simulink model "Microgrid_W"  (R2020a)
settings: Solver=ode15s  StartTime=0  StopTime=1440*1  MaxStep=1  RelTol=1e-3
libraries: simulink x4214, powerlib x685, simulink_extras x28, Microgrid_Library x18, powerlib_meascontrol x12
(part 1 of 48)
settings Model: Creator=burmesdani  LastModifiedBy=danie
settings SolverCC: ZeroCrossAlgorithm=Adaptive
settings DataIOCC: ReturnWorkspaceOutputs=off
settings DebuggingCC: MaxConsecutiveZCsMsg=none  ArithmeticOperatorsInVariantConditions=warning
settings SFSimCC: SimUseLocalCustomCode=off  CustomCodeUndefinedFunction=UseInterfaceOnly
settings RTWCC: RTWUseLocalCustomCode=off
settings CodeAppCC: StateflowObjectComments=on
settings SimscapeCC: SimscapeNormalizeSystem=off

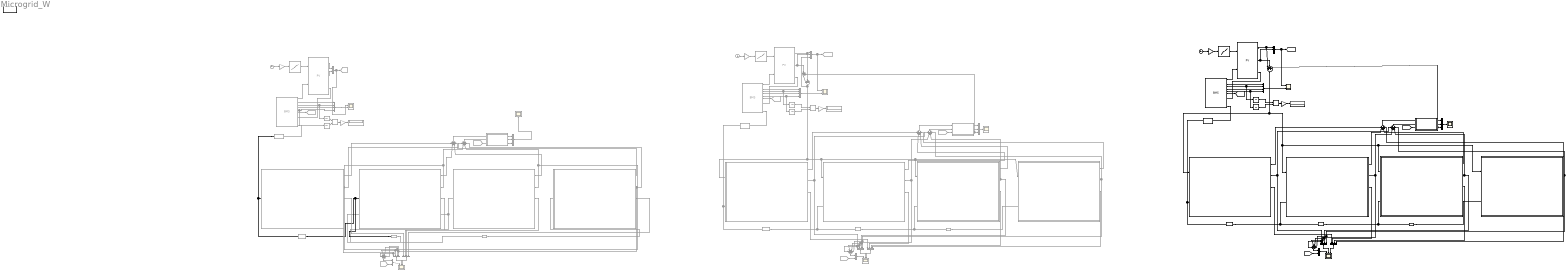
== system Microgrid_W ==
  note: Uncontrolled Microgrid
  note: Controlled Microgrid
  note: Controlled Microgrid
  1-D Lookup Table1 : Lookup_n-D  NumberOfTableDimensions=1  BreakpointsForDimension1=[ 0 1 2 3 4 5 6 7 8 9 10 11 12 13 14 15 16 17 18 19 20 21 22 23 24 25 26 27 28 29 30 31 32 33 34 35 36 37 38 39 40 41 42 43 44 45 46 47 48 49 50 51 52 53 54 55 56 57 58 59 60 61 62 63 64 65 66 67 68 69 70 71 72 73 74 75 76 77 78 79 80 81 82 83 84 85 86 87 88 89 90 91 92 93 94 95 96 97 98 99 100 101 102 103 104 105 106 107 108 109 110 111 112 113 114 115 116 117 118 119 120 121 122 123 124 125 126 127 128 129 130 131 132 133 134 135 136 137 138 139 140 141 142 143 144 145 146 147 148 149 150 151 152 153 154 155 156 157 158 159 160 161 162 163 164 165 166 167 ]  Table=|  InternalRulePriority=Speed  RndMeth=Simplest  InputSameDT=on
      | [ 0 0 0 0 0 0 0 0 24 102 216 265 347 180 457 139 14 0 0 0 0 0 0 0 0 0 0 0 0 0 0 3 102 438 606 521 454 674 419 211 67 0 0 0 0 0 0 0 0 0 0 0 0 0 0 0 20 56 105 60 86 80 111 69 23 0 0 0 0 0 0 0 0 0 0 0 0 0 0 0 20 59 207 329 494 326 573 325 86 0 0 0 0 0 0 0 0 0 0 0 0 0 0 3 79 461 545 698 753 631 556 256 120 0 0 0 0 0 0 0 0 0 0 0 0 0 0 0 23 289 555 185 105 97 116 180 25 0 0 0 0 0 0 0 0 0 0 0 0 0 0 0 26 66 128 161 217 251 160 48 40 0 0 0 0 0 0 0 
      | ]
  1-D Lookup Table2 : Lookup_n-D  Commented=on  NumberOfTableDimensions=1  BreakpointsForDimension1=[ 0 1 2 3 4 5 6 7 8 9 10 11 12 13 14 15 16 17 18 19 20 21 22 23 24 25 26 27 28 29 30 31 32 33 34 35 36 37 38 39 40 41 42 43 44 45 46 47 48 49 50 51 52 53 54 55 56 57 58 59 60 61 62 63 64 65 66 67 68 69 70 71 72 73 74 75 76 77 78 79 80 81 82 83 84 85 86 87 88 89 90 91 92 93 94 95 96 97 98 99 100 101 102 103 104 105 106 107 108 109 110 111 112 113 114 115 116 117 118 119 120 121 122 123 124 125 126 127 128 129 130 131 132 133 134 135 136 137 138 139 140 141 142 143 144 145 146 147 148 149 150 151 152 153 154 155 156 157 158 159 160 161 162 163 164 165 166 167 ]  Table=|  InternalRulePriority=Speed  RndMeth=Simplest  InputSameDT=on
      | [ 0 0 0 0 0 0 0 0 24 102 216 265 347 180 457 139 14 0 0 0 0 0 0 0 0 0 0 0 0 0 0 3 102 438 606 521 454 674 419 211 67 0 0 0 0 0 0 0 0 0 0 0 0 0 0 0 20 56 105 60 86 80 111 69 23 0 0 0 0 0 0 0 0 0 0 0 0 0 0 0 20 59 207 329 494 326 573 325 86 0 0 0 0 0 0 0 0 0 0 0 0 0 0 3 79 461 545 698 753 631 556 256 120 0 0 0 0 0 0 0 0 0 0 0 0 0 0 0 23 289 555 185 105 97 116 180 25 0 0 0 0 0 0 0 0 0 0 0 0 0 0 0 26 66 128 161 217 251 160 48 40 0 0 0 0 0 0 0 
      | ]
  1-D Lookup Table3 : Lookup_n-D  Commented=on  NumberOfTableDimensions=1  BreakpointsForDimension1=[ 0 1 2 3 4 5 6 7 8 9 10 11 12 13 14 15 16 17 18 19 20 21 22 23 24 25 26 27 28 29 30 31 32 33 34 35 36 37 38 39 40 41 42 43 44 45 46 47 48 49 50 51 52 53 54 55 56 57 58 59 60 61 62 63 64 65 66 67 68 69 70 71 72 73 74 75 76 77 78 79 80 81 82 83 84 85 86 87 88 89 90 91 92 93 94 95 96 97 98 99 100 101 102 103 104 105 106 107 108 109 110 111 112 113 114 115 116 117 118 119 120 121 122 123 124 125 126 127 128 129 130 131 132 133 134 135 136 137 138 139 140 141 142 143 144 145 146 147 148 149 150 151 152 153 154 155 156 157 158 159 160 161 162 163 164 165 166 167 ]  Table=|  InternalRulePriority=Speed  RndMeth=Simplest  InputSameDT=on
      | [ 0 0 0 0 0 0 0 0 24 102 216 265 347 180 457 139 14 0 0 0 0 0 0 0 0 0 0 0 0 0 0 3 102 438 606 521 454 674 419 211 67 0 0 0 0 0 0 0 0 0 0 0 0 0 0 0 20 56 105 60 86 80 111 69 23 0 0 0 0 0 0 0 0 0 0 0 0 0 0 0 20 59 207 329 494 326 573 325 86 0 0 0 0 0 0 0 0 0 0 0 0 0 0 3 79 461 545 698 753 631 556 256 120 0 0 0 0 0 0 0 0 0 0 0 0 0 0 0 23 289 555 185 105 97 116 180 25 0 0 0 0 0 0 0 0 0 0 0 0 0 0 0 26 66 128 161 217 251 160 48 40 0 0 0 0 0 0 0 
      | ]
  161m1 : Microgrid_Library/Line  l=161
  161m2 : Microgrid_Library/Line  Commented=on  l=161
  161m3 : Microgrid_Library/Line  Commented=on  l=161
  47m1 : Microgrid_Library/Line  l=47
  47m2 : Microgrid_Library/Line  Commented=on  l=47
  47m3 : Microgrid_Library/Line  Commented=on  l=47
  58m1 : Microgrid_Library/Line  l=58
  58m2 : Microgrid_Library/Line  Commented=on  l=58
  58m3 : Microgrid_Library/Line  Commented=on  l=58
  60m1 : Microgrid_Library/Line  l=60
  60m2 : Microgrid_Library/Line  Commented=on  l=60
  60m3 : Microgrid_Library/Line  Commented=on  l=60
  BMS1 : Microgrid_Library/BMS  v=240  c=460
  BMS2 : Microgrid_Library/BMS  Commented=on  v=240  c=460
  BMS3 : Microgrid_Library/BMS  Commented=on  v=240  c=460
  Clock1 : Clock
  Clock2 : Clock  Commented=on
  Clock3 : Clock  Commented=on
  Divide1 : Product  Inputs=*/
  Divide2 : Product  Commented=on  Inputs=*/
  Divide3 : Product  Commented=on  Inputs=*/
  From1 : From  Commented=on  GotoTag=PV
  From3 : From  Commented=on  GotoTag=bat_sup
  From4 : From  Commented=on  GotoTag=PV_MUX
  From5 : From  Commented=on  GotoTag=bat_sup
  Gain1 : Gain  Gain=1/60
  Gain2 : Gain  Gain=100
  Gain3 : Gain  Commented=on  Gain=1/60
  Gain4 : Gain  Commented=on  Gain=100
  Gain5 : Gain  Commented=on  Gain=1/60
  Gain6 : Gain  Commented=on  Gain=100
  Goto2 : Goto  Commented=on  GotoTag=PV
  Goto3 : Goto  Commented=on  GotoTag=bat_sup
  Goto4 : Goto  Commented=on  GotoTag=PV_MUX
  Goto5 : Goto  Commented=on  GotoTag=bat_sup
  House 2 W1 : Subsystem  AncestorBlock=Microgrid_Library/House 2 W  mask{V=240, t=60, K_L1_W=40, K_L1_On_1=63000, K_L1_Off_1=72600, K_L1_On_2=0, K_L1_Off_2=0, Dishwasher_W=1200, Dishwasher_On=72000, Fridge_W=150, T_Initial=1.9, T_Low=1, T_High=2.4, Jug_W=1500, Jug_On_1=25200, Jug_On_2=64200, Jug_On_3=0, Toaster_W=900, Toaster_On_1=23400, Toaster_On_2=27120, N_Elements=4, Oven_On_1=63600, Oven_Off_1=67200, Shower_On_a=21720, Shower_L_a=240, Shower_On_b=23640, Shower_L_b=300, Shower_On_c=0, Shower_L_c=0, K_L3_W=60, K_L3_On_1=21480, K_L3_Off_1=22140, K_L3_On_2=23580, K_L3_Off_2=24780, HW_W=2000, M=177, D=0.488, L=1.72, Ti=7, Ta=20, T_Low_WH=58, T_High_WH=61, Clock_1_W=5, Lamp_1_W=18, L1_On_1=79740, L1_Off_1=83040, L1_On_2=0, L1_Off_2=0, K_L4_W=24, K_L4_On_1=21000, K_L4_Off_1=27360, Clock_2_W=6, Lamp_2_W=24, L2_On_1=26820, L2_Off_1=29160, L2_On_2=73800, L2_Off_2=76800, K_L5_W=40, K_L5_On_1=28800, K_L5_Off_1=30240, K_L5_On_2=72300, K_L5_Off_2=83880, Phone_C_1_W=3, Phone_C_1_On_a=0, Phone_C_1_Off_a=35700, Phone_C_1_On_b=76800, Phone_C_1_Off_b=86400, Phone_C_2_W=7, Phone_C_2_On_a=0, Phone_C_2_Off_a=35760, Phone_C_2_On_b=76800, Phone_C_2_Off_b=86400, Phone_C_3_W=5, Phone_C_3_On_a=0, Phone_C_3_Off_a=35700, Phone_C_3_On_b=77040, Phone_C_3_Off_b=86400, Laptop_C_1_W=55, Laptop_C_1_On_a=76800, Laptop_C_1_Off_a=86400, Laptop_C_2_W=65, Laptop_C_2_On_a=0, Laptop_C_2_Off_a=28500, Laptop_C_2_On_b=77160, Laptop_C_2_Off_b=86400, Lamp_3_W=60, L3_On_1=21600, L3_Off_1=27000, L3_On_2=62760, L3_Off_2=83220, K_L6_W=60, K_L6_On_1=68400, K_L6_Off_1=70200, Heater_W=1800, Heater_On_1=62040, Heater_Off_1=68640, Stereo_W=100, Stereo_On_1=42480, Stereo_Off_1=58200, TV_W=500, TV_On_1=21900, TV_Off_1=26580, TV_On_2=63000, TV_Off_2=73200}
      mask prompts: V "Voltage"; t "Time"; K_L1_W "Light_1_W"; K_L1_On_1 "Light_1_On_a"; K_L1_Off_1 "Light_1_Off_a"; K_L1_On_2 "Light_1_On_b"; K_L1_Off_2 "Light_1_Off_b"; T_Initial "Fridge_Initial_Temp"; T_Low "Fridge_T_Low"; T_High "Fridge_T_High"; N_Elements "Oven_#_Elements"; Shower_L_a "Shower_Length_a"; Shower_L_b "Shower_Length_b"; Shower_L_c "Shower_Length_c"; K_L3_W "Light_3_W"; K_L3_On_1 "Light_3_On_a"; K_L3_Off_1 "Light_3_Off_a"; K_L3_On_2 "Light_3_On_b"; K_L3_Off_2 "Light_3_Off_b"; M "Mass of water"; D "HW_Diameter"; L "HW_Length"; Ti "Inlet Temp"; Ta "Ambient Temp"; L1_On_1 "Lamp_1_On_1"; L1_Off_1 "Lamp_1_Off_1"; L1_On_2 "Lamp_1_On_2"; L1_Off_2 "Lamp_1_Off_2"; K_L4_W "Light_4_W"; K_L4_On_1 "Light_4_On_a"; K_L4_Off_1 "Light_4_Off_a"; L2_On_1 "Lamp_2_On_1"; L2_Off_1 "Lamp_2_Off_1"; L2_On_2 "Lamp_2_On_2"; L2_Off_2 "Lamp_2_Off_2"; K_L5_W "Light_5_W"; K_L5_On_1 "Light_5_On_a"; K_L5_Off_1 "Light_5_Off_a"; K_L5_On_2 "Light_5_On_b"; K_L5_Off_2 "Light_5_Off_b"; L3_On_1 "Lamp_3_On_1"; L3_Off_1 "Lamp_3_Off_1"; L3_On_2 "Lamp_3_On_2"; L3_Off_2 "Lamp_3_Off_2"; K_L6_W "Light_6_W"; K_L6_On_1 "Light_6_On_a"; K_L6_Off_1 "Light_6_Off_a"
      mask DialogControl Container4 Prompt: House 1
      mask DialogControl Container10 Prompt: Kitchen
      mask DialogControl Container22 Prompt: Bathroom
      mask DialogControl Container20 Prompt: Bedroom 1
      mask DialogControl Container16 Prompt: Bedroom 2
      mask DialogControl Container11 Prompt: Lounge
      mask Display: image('house.jpg');
  House 2 W2 : Subsystem  Commented=on  AncestorBlock=Microgrid_Library/House 2 W  mask{V=240, t=60, K_L1_W=40, K_L1_On_1=63000, K_L1_Off_1=72600, K_L1_On_2=0, K_L1_Off_2=0, Dishwasher_W=1200, Dishwasher_On=72000, Fridge_W=150, T_Initial=1.9, T_Low=1, T_High=2.4, Jug_W=1500, Jug_On_1=25200, Jug_On_2=64200, Jug_On_3=0, Toaster_W=900, Toaster_On_1=23400, Toaster_On_2=27120, N_Elements=4, Oven_On_1=63600, Oven_Off_1=67200, Shower_On_a=21720, Shower_L_a=240, Shower_On_b=23640, Shower_L_b=300, Shower_On_c=0, Shower_L_c=0, K_L3_W=60, K_L3_On_1=21480, K_L3_Off_1=22140, K_L3_On_2=23580, K_L3_Off_2=24780, HW_W=2000, M=177, D=0.488, L=1.72, Ti=7, Ta=20, T_Low_WH=58, T_High_WH=61, Clock_1_W=5, Lamp_1_W=18, L1_On_1=79740, L1_Off_1=83040, L1_On_2=0, L1_Off_2=0, K_L4_W=24, K_L4_On_1=21000, K_L4_Off_1=27360, Clock_2_W=6, Lamp_2_W=24, L2_On_1=26820, L2_Off_1=29160, L2_On_2=73800, L2_Off_2=76800, K_L5_W=40, K_L5_On_1=28800, K_L5_Off_1=30240, K_L5_On_2=72300, K_L5_Off_2=83880, Phone_C_1_W=3, Phone_C_1_On_a=0, Phone_C_1_Off_a=35700, Phone_C_1_On_b=76800, Phone_C_1_Off_b=86400, Phone_C_2_W=7, Phone_C_2_On_a=0, Phone_C_2_Off_a=35760, Phone_C_2_On_b=76800, Phone_C_2_Off_b=86400, Phone_C_3_W=5, Phone_C_3_On_a=0, Phone_C_3_Off_a=35700, Phone_C_3_On_b=77040, Phone_C_3_Off_b=86400, Laptop_C_1_W=55, Laptop_C_1_On_a=76800, Laptop_C_1_Off_a=86400, Laptop_C_2_W=65, Laptop_C_2_On_a=0, Laptop_C_2_Off_a=28500, Laptop_C_2_On_b=77160, Laptop_C_2_Off_b=86400, Lamp_3_W=60, L3_On_1=21600, L3_Off_1=27000, L3_On_2=62760, L3_Off_2=83220, K_L6_W=60, K_L6_On_1=68400, K_L6_Off_1=70200, Heater_W=1800, Heater_On_1=62040, Heater_Off_1=68640, Stereo_W=100, Stereo_On_1=42480, Stereo_Off_1=58200, TV_W=500, TV_On_1=21900, TV_Off_1=26580, TV_On_2=63000, TV_Off_2=73200}
      mask prompts: V "Voltage"; t "Time"; K_L1_W "Light_1_W"; K_L1_On_1 "Light_1_On_a"; K_L1_Off_1 "Light_1_Off_a"; K_L1_On_2 "Light_1_On_b"; K_L1_Off_2 "Light_1_Off_b"; T_Initial "Fridge_Initial_Temp"; T_Low "Fridge_T_Low"; T_High "Fridge_T_High"; N_Elements "Oven_#_Elements"; Shower_L_a "Shower_Length_a"; Shower_L_b "Shower_Length_b"; Shower_L_c "Shower_Length_c"; K_L3_W "Light_3_W"; K_L3_On_1 "Light_3_On_a"; K_L3_Off_1 "Light_3_Off_a"; K_L3_On_2 "Light_3_On_b"; K_L3_Off_2 "Light_3_Off_b"; M "Mass of water"; D "HW_Diameter"; L "HW_Length"; Ti "Inlet Temp"; Ta "Ambient Temp"; L1_On_1 "Lamp_1_On_1"; L1_Off_1 "Lamp_1_Off_1"; L1_On_2 "Lamp_1_On_2"; L1_Off_2 "Lamp_1_Off_2"; K_L4_W "Light_4_W"; K_L4_On_1 "Light_4_On_a"; K_L4_Off_1 "Light_4_Off_a"; L2_On_1 "Lamp_2_On_1"; L2_Off_1 "Lamp_2_Off_1"; L2_On_2 "Lamp_2_On_2"; L2_Off_2 "Lamp_2_Off_2"; K_L5_W "Light_5_W"; K_L5_On_1 "Light_5_On_a"; K_L5_Off_1 "Light_5_Off_a"; K_L5_On_2 "Light_5_On_b"; K_L5_Off_2 "Light_5_Off_b"; L3_On_1 "Lamp_3_On_1"; L3_Off_1 "Lamp_3_Off_1"; L3_On_2 "Lamp_3_On_2"; L3_Off_2 "Lamp_3_Off_2"; K_L6_W "Light_6_W"; K_L6_On_1 "Light_6_On_a"; K_L6_Off_1 "Light_6_Off_a"
      mask DialogControl Container4 Prompt: House 1
      mask DialogControl Container10 Prompt: Kitchen
      mask DialogControl Container22 Prompt: Bathroom
      mask DialogControl Container20 Prompt: Bedroom 1
      mask DialogControl Container16 Prompt: Bedroom 2
      mask DialogControl Container11 Prompt: Lounge
      mask Display: image('house.jpg');
  House 2 W3 : Subsystem  Commented=on  AncestorBlock=Microgrid_Library/House 2 W  mask{V=240, t=60, K_L1_W=40, K_L1_On_1=63000, K_L1_Off_1=72600, K_L1_On_2=0, K_L1_Off_2=0, Dishwasher_W=1200, Dishwasher_On=72000, Fridge_W=150, T_Initial=1.9, T_Low=1, T_High=2.4, Jug_W=1500, Jug_On_1=25200, Jug_On_2=64200, Jug_On_3=0, Toaster_W=900, Toaster_On_1=23400, Toaster_On_2=27120, N_Elements=4, Oven_On_1=63600, Oven_Off_1=67200, Shower_On_a=21720, Shower_L_a=240, Shower_On_b=23640, Shower_L_b=300, Shower_On_c=0, Shower_L_c=0, K_L3_W=60, K_L3_On_1=21480, K_L3_Off_1=22140, K_L3_On_2=23580, K_L3_Off_2=24780, HW_W=2000, M=177, D=0.488, L=1.72, Ti=7, Ta=20, T_Low_WH=58, T_High_WH=61, Clock_1_W=5, Lamp_1_W=18, L1_On_1=79740, L1_Off_1=83040, L1_On_2=0, L1_Off_2=0, K_L4_W=24, K_L4_On_1=21000, K_L4_Off_1=27360, Clock_2_W=6, Lamp_2_W=24, L2_On_1=26820, L2_Off_1=29160, L2_On_2=73800, L2_Off_2=76800, K_L5_W=40, K_L5_On_1=28800, K_L5_Off_1=30240, K_L5_On_2=72300, K_L5_Off_2=83880, Phone_C_1_W=3, Phone_C_1_On_a=0, Phone_C_1_Off_a=35700, Phone_C_1_On_b=76800, Phone_C_1_Off_b=86400, Phone_C_2_W=7, Phone_C_2_On_a=0, Phone_C_2_Off_a=35760, Phone_C_2_On_b=76800, Phone_C_2_Off_b=86400, Phone_C_3_W=5, Phone_C_3_On_a=0, Phone_C_3_Off_a=35700, Phone_C_3_On_b=77040, Phone_C_3_Off_b=86400, Laptop_C_1_W=55, Laptop_C_1_On_a=76800, Laptop_C_1_Off_a=86400, Laptop_C_2_W=65, Laptop_C_2_On_a=0, Laptop_C_2_Off_a=28500, Laptop_C_2_On_b=77160, Laptop_C_2_Off_b=86400, Lamp_3_W=60, L3_On_1=21600, L3_Off_1=27000, L3_On_2=62760, L3_Off_2=83220, K_L6_W=60, K_L6_On_1=68400, K_L6_Off_1=70200, Heater_W=1800, Heater_On_1=62040, Heater_Off_1=68640, Stereo_W=100, Stereo_On_1=42480, Stereo_Off_1=58200, TV_W=500, TV_On_1=21900, TV_Off_1=26580, TV_On_2=63000, TV_Off_2=73200}
      mask prompts: V "Voltage"; t "Time"; K_L1_W "Light_1_W"; K_L1_On_1 "Light_1_On_a"; K_L1_Off_1 "Light_1_Off_a"; K_L1_On_2 "Light_1_On_b"; K_L1_Off_2 "Light_1_Off_b"; T_Initial "Fridge_Initial_Temp"; T_Low "Fridge_T_Low"; T_High "Fridge_T_High"; N_Elements "Oven_#_Elements"; Shower_L_a "Shower_Length_a"; Shower_L_b "Shower_Length_b"; Shower_L_c "Shower_Length_c"; K_L3_W "Light_3_W"; K_L3_On_1 "Light_3_On_a"; K_L3_Off_1 "Light_3_Off_a"; K_L3_On_2 "Light_3_On_b"; K_L3_Off_2 "Light_3_Off_b"; M "Mass of water"; D "HW_Diameter"; L "HW_Length"; Ti "Inlet Temp"; Ta "Ambient Temp"; L1_On_1 "Lamp_1_On_1"; L1_Off_1 "Lamp_1_Off_1"; L1_On_2 "Lamp_1_On_2"; L1_Off_2 "Lamp_1_Off_2"; K_L4_W "Light_4_W"; K_L4_On_1 "Light_4_On_a"; K_L4_Off_1 "Light_4_Off_a"; L2_On_1 "Lamp_2_On_1"; L2_Off_1 "Lamp_2_Off_1"; L2_On_2 "Lamp_2_On_2"; L2_Off_2 "Lamp_2_Off_2"; K_L5_W "Light_5_W"; K_L5_On_1 "Light_5_On_a"; K_L5_Off_1 "Light_5_Off_a"; K_L5_On_2 "Light_5_On_b"; K_L5_Off_2 "Light_5_Off_b"; L3_On_1 "Lamp_3_On_1"; L3_Off_1 "Lamp_3_Off_1"; L3_On_2 "Lamp_3_On_2"; L3_Off_2 "Lamp_3_Off_2"; K_L6_W "Light_6_W"; K_L6_On_1 "Light_6_On_a"; K_L6_Off_1 "Light_6_Off_a"
      mask DialogControl Container4 Prompt: House 1
      mask DialogControl Container10 Prompt: Kitchen
      mask DialogControl Container22 Prompt: Bathroom
      mask DialogControl Container20 Prompt: Bedroom 1
      mask DialogControl Container16 Prompt: Bedroom 2
      mask DialogControl Container11 Prompt: Lounge
      mask Display: image('house.jpg');
  House 3 W1 : Subsystem  AncestorBlock=Microgrid_Library/House 3 W  mask{V=240, t=60, K_L1_W=24, K_L1_On_1=21600, K_L1_Off_1=26580, K_L1_On_2=63000, K_L1_Off_2=68400, K_L2_W=60, K_L2_On_1=63000, K_L2_Off_1=68400, Fridge_W=200, T_Initial=1.5, T_Low=1.5, T_High=2.65, Jug_W=2000, Jug_On_1=21720, Jug_On_2=43560, Jug_On_3=73800, Toaster_W=1200, Toaster_On_1=25260, Toaster_On_2=28920, N_Elements=1, Oven_On_1=58680, Oven_Off_1=68760, Shower_On_a=70440, Shower_L_a=360, Shower_On_b=76740, Shower_L_b=180, Shower_On_c=81000, Shower_L_c=180, K_L3_W=80, K_L3_On_1=70200, K_L3_Off_1=70800, K_L3_On_2=76320, K_L3_Off_2=81300, HW_W=3000, M=250, D=0.58, L=1.56, Ti=7, Ta=20, T_Low_WH=59, T_High_WH=61, Clock_1_W=6, Lamp_1_W=18, L1_On_1=71400, L1_Off_1=81120, L1_On_2=0, L1_Off_2=0, K_L4_W=60, K_L4_On_1=69600, K_L4_Off_1=71400, Clock_2_W=4, Lamp_2_W=24, L2_On_1=84120, L2_Off_1=86880, L2_On_2=0, L2_Off_2=0, K_L5_W=40, K_L5_On_1=25320, K_L5_Off_1=28980, K_L5_On_2=81000, K_L5_Off_2=84180, Phone_C_1_W=7, Phone_C_1_On_a=0, Phone_C_1_Off_a=27300, Phone_C_1_On_b=79200, Phone_C_1_Off_b=86400, Phone_C_2_W=6, Phone_C_2_On_a=0, Phone_C_2_Off_a=27300, Phone_C_2_On_b=79200, Phone_C_2_Off_b=86400, Phone_C_3_W=5, Phone_C_3_On_a=0, Phone_C_3_Off_a=0, Phone_C_3_On_b=0, Phone_C_3_Off_b=0, Laptop_C_1_W=1, Laptop_C_1_On_a=0, Laptop_C_1_Off_a=0, Laptop_C_2_W=45, Laptop_C_2_On_a=0, Laptop_C_2_Off_a=6000, Laptop_C_2_On_b=66600, Laptop_C_2_Off_b=86400, Lamp_3_W=40, L3_On_1=24900, L3_Off_1=30600, L3_On_2=72000, L3_Off_2=81000, K_L6_W=60, K_L6_On_1=68760, K_L6_Off_1=71520, Heater_W=1500, Heater_On_1=64800, Heater_Off_1=78000, Stereo_W=1, Stereo_On_1=0, Stereo_Off_1=0, TV_W=150, TV_On_1=25200, TV_Off_1=28800, TV_On_2=72240, TV_Off_2=81000}
      mask prompts: V "Voltage"; t "Time"; K_L1_W "Light_1_W"; K_L1_On_1 "Light_1_On_a"; K_L1_Off_1 "Light_1_Off_a"; K_L1_On_2 "Light_1_On_b"; K_L1_Off_2 "Light_1_Off_b"; K_L2_W "Light_2_W"; K_L2_On_1 "Light_2_On_a"; K_L2_Off_1 "Light_2_Off_a"; T_Initial "Fridge_Initial_Temp"; T_Low "Fridge_T_Low"; T_High "Fridge_T_High"; N_Elements "Oven_#_Elements"; Shower_L_a "Shower_Length_a"; Shower_L_b "Shower_Length_b"; Shower_L_c "Shower_Length_c"; K_L3_W "Light_3_W"; K_L3_On_1 "Light_3_On_a"; K_L3_Off_1 "Light_3_Off_a"; K_L3_On_2 "Light_3_On_b"; K_L3_Off_2 "Light_3_Off_b"; M "Mass of water"; D "HW_Diameter"; L "HW_Length"; Ti "Inlet Temp"; Ta "Ambient Temp"; L1_On_1 "Lamp_1_On_1"; L1_Off_1 "Lamp_1_Off_1"; L1_On_2 "Lamp_1_On_2"; L1_Off_2 "Lamp_1_Off_2"; K_L4_W "Light_4_W"; K_L4_On_1 "Light_4_On_a"; K_L4_Off_1 "Light_4_Off_a"; L2_On_1 "Lamp_2_On_1"; L2_Off_1 "Lamp_2_Off_1"; L2_On_2 "Lamp_2_On_2"; L2_Off_2 "Lamp_2_Off_2"; K_L5_W "Light_5_W"; K_L5_On_1 "Light_5_On_a"; K_L5_Off_1 "Light_5_Off_a"; K_L5_On_2 "Light_5_On_b"; K_L5_Off_2 "Light_5_Off_b"; L3_On_1 "Lamp_3_On_1"; L3_Off_1 "Lamp_3_Off_1"; L3_On_2 "Lamp_3_On_2"; L3_Off_2 "Lamp_3_Off_2"; K_L6_W "Light_6_W"; K_L6_On_1 "Light_6_On_a"; K_L6_Off_1 "Light_6_Off_a"
      mask DialogControl Container4 Prompt: House 1
      mask DialogControl Container10 Prompt: Kitchen
      mask DialogControl Container22 Prompt: Bathroom
      mask DialogControl Container20 Prompt: Bedroom 1
      mask DialogControl Container16 Prompt: Bedroom 2
      mask DialogControl Container11 Prompt: Lounge
      mask Display: image('house.jpg');
  House 3 W2 : Subsystem  Commented=on  AncestorBlock=Microgrid_Library/House 3 W  mask{V=240, t=60, K_L1_W=24, K_L1_On_1=21600, K_L1_Off_1=26580, K_L1_On_2=63000, K_L1_Off_2=68400, K_L2_W=60, K_L2_On_1=63000, K_L2_Off_1=68400, Fridge_W=200, T_Initial=1.5, T_Low=1.5, T_High=2.65, Jug_W=2000, Jug_On_1=21720, Jug_On_2=43560, Jug_On_3=73800, Toaster_W=1200, Toaster_On_1=25260, Toaster_On_2=28920, N_Elements=1, Oven_On_1=58680, Oven_Off_1=68760, Shower_On_a=70440, Shower_L_a=360, Shower_On_b=76740, Shower_L_b=180, Shower_On_c=81000, Shower_L_c=180, K_L3_W=80, K_L3_On_1=70200, K_L3_Off_1=70800, K_L3_On_2=76320, K_L3_Off_2=81300, HW_W=3000, M=250, D=0.58, L=1.56, Ti=7, Ta=20, T_Low_WH=59, T_High_WH=61, Clock_1_W=6, Lamp_1_W=18, L1_On_1=71400, L1_Off_1=81120, L1_On_2=0, L1_Off_2=0, K_L4_W=60, K_L4_On_1=69600, K_L4_Off_1=71400, Clock_2_W=4, Lamp_2_W=24, L2_On_1=84120, L2_Off_1=86880, L2_On_2=0, L2_Off_2=0, K_L5_W=40, K_L5_On_1=25320, K_L5_Off_1=28980, K_L5_On_2=81000, K_L5_Off_2=84180, Phone_C_1_W=7, Phone_C_1_On_a=0, Phone_C_1_Off_a=27300, Phone_C_1_On_b=79200, Phone_C_1_Off_b=86400, Phone_C_2_W=6, Phone_C_2_On_a=0, Phone_C_2_Off_a=27300, Phone_C_2_On_b=79200, Phone_C_2_Off_b=86400, Phone_C_3_W=5, Phone_C_3_On_a=0, Phone_C_3_Off_a=0, Phone_C_3_On_b=0, Phone_C_3_Off_b=0, Laptop_C_1_W=1, Laptop_C_1_On_a=0, Laptop_C_1_Off_a=0, Laptop_C_2_W=45, Laptop_C_2_On_a=0, Laptop_C_2_Off_a=6000, Laptop_C_2_On_b=66600, Laptop_C_2_Off_b=86400, Lamp_3_W=40, L3_On_1=24900, L3_Off_1=30600, L3_On_2=72000, L3_Off_2=81000, K_L6_W=60, K_L6_On_1=68760, K_L6_Off_1=71520, Heater_W=1500, Heater_On_1=64800, Heater_Off_1=78000, Stereo_W=1, Stereo_On_1=0, Stereo_Off_1=0, TV_W=150, TV_On_1=25200, TV_Off_1=28800, TV_On_2=72240, TV_Off_2=81000}
      mask prompts: V "Voltage"; t "Time"; K_L1_W "Light_1_W"; K_L1_On_1 "Light_1_On_a"; K_L1_Off_1 "Light_1_Off_a"; K_L1_On_2 "Light_1_On_b"; K_L1_Off_2 "Light_1_Off_b"; K_L2_W "Light_2_W"; K_L2_On_1 "Light_2_On_a"; K_L2_Off_1 "Light_2_Off_a"; T_Initial "Fridge_Initial_Temp"; T_Low "Fridge_T_Low"; T_High "Fridge_T_High"; N_Elements "Oven_#_Elements"; Shower_L_a "Shower_Length_a"; Shower_L_b "Shower_Length_b"; Shower_L_c "Shower_Length_c"; K_L3_W "Light_3_W"; K_L3_On_1 "Light_3_On_a"; K_L3_Off_1 "Light_3_Off_a"; K_L3_On_2 "Light_3_On_b"; K_L3_Off_2 "Light_3_Off_b"; M "Mass of water"; D "HW_Diameter"; L "HW_Length"; Ti "Inlet Temp"; Ta "Ambient Temp"; L1_On_1 "Lamp_1_On_1"; L1_Off_1 "Lamp_1_Off_1"; L1_On_2 "Lamp_1_On_2"; L1_Off_2 "Lamp_1_Off_2"; K_L4_W "Light_4_W"; K_L4_On_1 "Light_4_On_a"; K_L4_Off_1 "Light_4_Off_a"; L2_On_1 "Lamp_2_On_1"; L2_Off_1 "Lamp_2_Off_1"; L2_On_2 "Lamp_2_On_2"; L2_Off_2 "Lamp_2_Off_2"; K_L5_W "Light_5_W"; K_L5_On_1 "Light_5_On_a"; K_L5_Off_1 "Light_5_Off_a"; K_L5_On_2 "Light_5_On_b"; K_L5_Off_2 "Light_5_Off_b"; L3_On_1 "Lamp_3_On_1"; L3_Off_1 "Lamp_3_Off_1"; L3_On_2 "Lamp_3_On_2"; L3_Off_2 "Lamp_3_Off_2"; K_L6_W "Light_6_W"; K_L6_On_1 "Light_6_On_a"; K_L6_Off_1 "Light_6_Off_a"
      mask DialogControl Container4 Prompt: House 1
      mask DialogControl Container10 Prompt: Kitchen
      mask DialogControl Container22 Prompt: Bathroom
      mask DialogControl Container20 Prompt: Bedroom 1
      mask DialogControl Container16 Prompt: Bedroom 2
      mask DialogControl Container11 Prompt: Lounge
      mask Display: image('house.jpg');
  House 3 W3 : Subsystem  Commented=on  AncestorBlock=Microgrid_Library/House 3 W  mask{V=240, t=60, K_L1_W=24, K_L1_On_1=21600, K_L1_Off_1=26580, K_L1_On_2=63000, K_L1_Off_2=68400, K_L2_W=60, K_L2_On_1=63000, K_L2_Off_1=68400, Fridge_W=200, T_Initial=1.5, T_Low=1.5, T_High=2.65, Jug_W=2000, Jug_On_1=21720, Jug_On_2=43560, Jug_On_3=73800, Toaster_W=1200, Toaster_On_1=25260, Toaster_On_2=28920, N_Elements=1, Oven_On_1=58680, Oven_Off_1=68760, Shower_On_a=70440, Shower_L_a=360, Shower_On_b=76740, Shower_L_b=180, Shower_On_c=81000, Shower_L_c=180, K_L3_W=80, K_L3_On_1=70200, K_L3_Off_1=70800, K_L3_On_2=76320, K_L3_Off_2=81300, HW_W=3000, M=250, D=0.58, L=1.56, Ti=7, Ta=20, T_Low_WH=59, T_High_WH=61, Clock_1_W=6, Lamp_1_W=18, L1_On_1=71400, L1_Off_1=81120, L1_On_2=0, L1_Off_2=0, K_L4_W=60, K_L4_On_1=69600, K_L4_Off_1=71400, Clock_2_W=4, Lamp_2_W=24, L2_On_1=84120, L2_Off_1=86880, L2_On_2=0, L2_Off_2=0, K_L5_W=40, K_L5_On_1=25320, K_L5_Off_1=28980, K_L5_On_2=81000, K_L5_Off_2=84180, Phone_C_1_W=7, Phone_C_1_On_a=0, Phone_C_1_Off_a=27300, Phone_C_1_On_b=79200, Phone_C_1_Off_b=86400, Phone_C_2_W=6, Phone_C_2_On_a=0, Phone_C_2_Off_a=27300, Phone_C_2_On_b=79200, Phone_C_2_Off_b=86400, Phone_C_3_W=5, Phone_C_3_On_a=0, Phone_C_3_Off_a=0, Phone_C_3_On_b=0, Phone_C_3_Off_b=0, Laptop_C_1_W=1, Laptop_C_1_On_a=0, Laptop_C_1_Off_a=0, Laptop_C_2_W=45, Laptop_C_2_On_a=0, Laptop_C_2_Off_a=6000, Laptop_C_2_On_b=66600, Laptop_C_2_Off_b=86400, Lamp_3_W=40, L3_On_1=24900, L3_Off_1=30600, L3_On_2=72000, L3_Off_2=81000, K_L6_W=60, K_L6_On_1=68760, K_L6_Off_1=71520, Heater_W=1500, Heater_On_1=64800, Heater_Off_1=78000, Stereo_W=1, Stereo_On_1=0, Stereo_Off_1=0, TV_W=150, TV_On_1=25200, TV_Off_1=28800, TV_On_2=72240, TV_Off_2=81000}
      mask prompts: V "Voltage"; t "Time"; K_L1_W "Light_1_W"; K_L1_On_1 "Light_1_On_a"; K_L1_Off_1 "Light_1_Off_a"; K_L1_On_2 "Light_1_On_b"; K_L1_Off_2 "Light_1_Off_b"; K_L2_W "Light_2_W"; K_L2_On_1 "Light_2_On_a"; K_L2_Off_1 "Light_2_Off_a"; T_Initial "Fridge_Initial_Temp"; T_Low "Fridge_T_Low"; T_High "Fridge_T_High"; N_Elements "Oven_#_Elements"; Shower_L_a "Shower_Length_a"; Shower_L_b "Shower_Length_b"; Shower_L_c "Shower_Length_c"; K_L3_W "Light_3_W"; K_L3_On_1 "Light_3_On_a"; K_L3_Off_1 "Light_3_Off_a"; K_L3_On_2 "Light_3_On_b"; K_L3_Off_2 "Light_3_Off_b"; M "Mass of water"; D "HW_Diameter"; L "HW_Length"; Ti "Inlet Temp"; Ta "Ambient Temp"; L1_On_1 "Lamp_1_On_1"; L1_Off_1 "Lamp_1_Off_1"; L1_On_2 "Lamp_1_On_2"; L1_Off_2 "Lamp_1_Off_2"; K_L4_W "Light_4_W"; K_L4_On_1 "Light_4_On_a"; K_L4_Off_1 "Light_4_Off_a"; L2_On_1 "Lamp_2_On_1"; L2_Off_1 "Lamp_2_Off_1"; L2_On_2 "Lamp_2_On_2"; L2_Off_2 "Lamp_2_Off_2"; K_L5_W "Light_5_W"; K_L5_On_1 "Light_5_On_a"; K_L5_Off_1 "Light_5_Off_a"; K_L5_On_2 "Light_5_On_b"; K_L5_Off_2 "Light_5_Off_b"; L3_On_1 "Lamp_3_On_1"; L3_Off_1 "Lamp_3_Off_1"; L3_On_2 "Lamp_3_On_2"; L3_Off_2 "Lamp_3_Off_2"; K_L6_W "Light_6_W"; K_L6_On_1 "Light_6_On_a"; K_L6_Off_1 "Light_6_Off_a"
      mask DialogControl Container4 Prompt: House 1
      mask DialogControl Container10 Prompt: Kitchen
      mask DialogControl Container22 Prompt: Bathroom
      mask DialogControl Container20 Prompt: Bedroom 1
      mask DialogControl Container16 Prompt: Bedroom 2
      mask DialogControl Container11 Prompt: Lounge
      mask Display: image('house.jpg');
  House 4 W1 : Subsystem  AncestorBlock=Microgrid_Library/House 4 W  mask{V=240, t=60, K_L1_W=60, K_L1_On_1=69180, K_L1_Off_1=70200, K_L1_On_2=0, K_L1_Off_2=0, K_L2_W=1, K_L2_On_1=0, K_L2_Off_1=0, Fridge_W=150, T_Initial=1, T_Low=1, T_High=3.6, Jug_W=1800, Jug_On_1=23760, Jug_On_2=79800, Jug_On_3=0, Toaster_W=1000, Toaster_On_1=21600, Toaster_On_2=0, N_Elements=2, Oven_On_1=69240, Oven_Off_1=70140, Shower_On_a=20040, Shower_L_a=180, Shower_On_b=0, Shower_L_b=0, Shower_On_c=0, Shower_L_c=0, K_L3_W=40, K_L3_On_1=19800, K_L3_Off_1=20400, K_L3_On_2=0, K_L3_Off_2=0, HW_W=2000, M=88, D=0.488, L=0.955, Ti=7, Ta=20, T_Low_WH=55, T_High_WH=59.5, Clock_1_W=0, Lamp_1_W=1, L1_On_1=0, L1_Off_1=0, L1_On_2=0, L1_Off_2=0, K_L4_W=1, K_L4_On_1=0, K_L4_Off_1=0, Clock_2_W=4, Lamp_2_W=40, L2_On_1=19680, L2_Off_1=21600, L2_On_2=82800, L2_Off_2=84600, K_L5_W=1, K_L5_On_1=0, K_L5_Off_1=0, K_L5_On_2=0, K_L5_Off_2=0, Phone_C_1_W=5, Phone_C_1_On_a=0, Phone_C_1_Off_a=27300, Phone_C_1_On_b=79200, Phone_C_1_Off_b=86400, Phone_C_2_W=0, Phone_C_2_On_a=0, Phone_C_2_Off_a=0, Phone_C_2_On_b=0, Phone_C_2_Off_b=0, Phone_C_3_W=0, Phone_C_3_On_a=0, Phone_C_3_Off_a=0, Phone_C_3_On_b=0, Phone_C_3_Off_b=0, Laptop_C_1_W=35, Laptop_C_1_On_a=63900, Laptop_C_1_Off_a=75600, Laptop_C_2_W=65, Laptop_C_2_On_a=0, Laptop_C_2_Off_a=21600, Laptop_C_2_On_b=66600, Laptop_C_2_Off_b=86400, Lamp_3_W=18, L3_On_1=66000, L3_Off_1=82800, L3_On_2=0, L3_Off_2=0, K_L6_W=40, K_L6_On_1=63000, K_L6_Off_1=66000, Heater_W=2000, Heater_On_1=65100, Heater_Off_1=82200, Stereo_W=100, Stereo_On_1=68640, Stereo_Off_1=70740, TV_W=300, TV_On_1=70800, TV_Off_1=82800, TV_On_2=0, TV_Off_2=0}
      mask prompts: V "Voltage"; t "Time"; K_L1_W "Light_1_W"; K_L1_On_1 "Light_1_On_a"; K_L1_Off_1 "Light_1_Off_a"; K_L1_On_2 "Light_1_On_b"; K_L1_Off_2 "Light_1_Off_b"; K_L2_W "Light_2_W"; K_L2_On_1 "Light_2_On_a"; K_L2_Off_1 "Light_2_Off_a"; T_Initial "Fridge_Initial_Temp"; T_Low "Fridge_T_Low"; T_High "Fridge_T_High"; N_Elements "Oven_#_Elements"; Shower_L_a "Shower_Length_a"; Shower_L_b "Shower_Length_b"; Shower_L_c "Shower_Length_c"; K_L3_W "Light_3_W"; K_L3_On_1 "Light_3_On_a"; K_L3_Off_1 "Light_3_Off_a"; K_L3_On_2 "Light_3_On_b"; K_L3_Off_2 "Light_3_Off_b"; M "Mass of water"; D "HW_Diameter"; L "HW_Length"; Ti "Inlet Temp"; Ta "Ambient Temp"; L1_On_1 "Lamp_1_On_1"; L1_Off_1 "Lamp_1_Off_1"; L1_On_2 "Lamp_1_On_2"; L1_Off_2 "Lamp_1_Off_2"; K_L4_W "Light_4_W"; K_L4_On_1 "Light_4_On_a"; K_L4_Off_1 "Light_4_Off_a"; L2_On_1 "Lamp_2_On_1"; L2_Off_1 "Lamp_2_Off_1"; L2_On_2 "Lamp_2_On_2"; L2_Off_2 "Lamp_2_Off_2"; K_L5_W "Light_5_W"; K_L5_On_1 "Light_5_On_a"; K_L5_Off_1 "Light_5_Off_a"; K_L5_On_2 "Light_5_On_b"; K_L5_Off_2 "Light_5_Off_b"; L3_On_1 "Lamp_3_On_1"; L3_Off_1 "Lamp_3_Off_1"; L3_On_2 "Lamp_3_On_2"; L3_Off_2 "Lamp_3_Off_2"; K_L6_W "Light_6_W"; K_L6_On_1 "Light_6_On_a"; K_L6_Off_1 "Light_6_Off_a"
      mask DialogControl Container4 Prompt: House 1
      mask DialogControl Container10 Prompt: Kitchen
      mask DialogControl Container22 Prompt: Bathroom
      mask DialogControl Container20 Prompt: Bedroom 1
      mask DialogControl Container16 Prompt: Bedroom 2
      mask DialogControl Container11 Prompt: Lounge
      mask Display: image('house.jpg');
  House 4 W2 : Subsystem  Commented=on  AncestorBlock=Microgrid_Library/House 4 W  mask{V=240, t=60, K_L1_W=60, K_L1_On_1=69180, K_L1_Off_1=70200, K_L1_On_2=0, K_L1_Off_2=0, K_L2_W=1, K_L2_On_1=0, K_L2_Off_1=0, Fridge_W=150, T_Initial=1, T_Low=1, T_High=3.6, Jug_W=1800, Jug_On_1=23760, Jug_On_2=79800, Jug_On_3=0, Toaster_W=1000, Toaster_On_1=21600, Toaster_On_2=0, N_Elements=2, Oven_On_1=69240, Oven_Off_1=70140, Shower_On_a=20040, Shower_L_a=180, Shower_On_b=0, Shower_L_b=0, Shower_On_c=0, Shower_L_c=0, K_L3_W=40, K_L3_On_1=19800, K_L3_Off_1=20400, K_L3_On_2=0, K_L3_Off_2=0, HW_W=2000, M=88, D=0.488, L=0.955, Ti=7, Ta=20, T_Low_WH=55, T_High_WH=59.5, Clock_1_W=0, Lamp_1_W=1, L1_On_1=0, L1_Off_1=0, L1_On_2=0, L1_Off_2=0, K_L4_W=1, K_L4_On_1=0, K_L4_Off_1=0, Clock_2_W=4, Lamp_2_W=40, L2_On_1=19680, L2_Off_1=21600, L2_On_2=82800, L2_Off_2=84600, K_L5_W=1, K_L5_On_1=0, K_L5_Off_1=0, K_L5_On_2=0, K_L5_Off_2=0, Phone_C_1_W=5, Phone_C_1_On_a=0, Phone_C_1_Off_a=27300, Phone_C_1_On_b=79200, Phone_C_1_Off_b=86400, Phone_C_2_W=0, Phone_C_2_On_a=0, Phone_C_2_Off_a=0, Phone_C_2_On_b=0, Phone_C_2_Off_b=0, Phone_C_3_W=0, Phone_C_3_On_a=0, Phone_C_3_Off_a=0, Phone_C_3_On_b=0, Phone_C_3_Off_b=0, Laptop_C_1_W=35, Laptop_C_1_On_a=63900, Laptop_C_1_Off_a=75600, Laptop_C_2_W=65, Laptop_C_2_On_a=0, Laptop_C_2_Off_a=21600, Laptop_C_2_On_b=66600, Laptop_C_2_Off_b=86400, Lamp_3_W=18, L3_On_1=66000, L3_Off_1=82800, L3_On_2=0, L3_Off_2=0, K_L6_W=40, K_L6_On_1=63000, K_L6_Off_1=66000, Heater_W=2000, Heater_On_1=65100, Heater_Off_1=82200, Stereo_W=100, Stereo_On_1=68640, Stereo_Off_1=70740, TV_W=300, TV_On_1=70800, TV_Off_1=82800, TV_On_2=0, TV_Off_2=0}
      mask prompts: V "Voltage"; t "Time"; K_L1_W "Light_1_W"; K_L1_On_1 "Light_1_On_a"; K_L1_Off_1 "Light_1_Off_a"; K_L1_On_2 "Light_1_On_b"; K_L1_Off_2 "Light_1_Off_b"; K_L2_W "Light_2_W"; K_L2_On_1 "Light_2_On_a"; K_L2_Off_1 "Light_2_Off_a"; T_Initial "Fridge_Initial_Temp"; T_Low "Fridge_T_Low"; T_High "Fridge_T_High"; N_Elements "Oven_#_Elements"; Shower_L_a "Shower_Length_a"; Shower_L_b "Shower_Length_b"; Shower_L_c "Shower_Length_c"; K_L3_W "Light_3_W"; K_L3_On_1 "Light_3_On_a"; K_L3_Off_1 "Light_3_Off_a"; K_L3_On_2 "Light_3_On_b"; K_L3_Off_2 "Light_3_Off_b"; M "Mass of water"; D "HW_Diameter"; L "HW_Length"; Ti "Inlet Temp"; Ta "Ambient Temp"; L1_On_1 "Lamp_1_On_1"; L1_Off_1 "Lamp_1_Off_1"; L1_On_2 "Lamp_1_On_2"; L1_Off_2 "Lamp_1_Off_2"; K_L4_W "Light_4_W"; K_L4_On_1 "Light_4_On_a"; K_L4_Off_1 "Light_4_Off_a"; L2_On_1 "Lamp_2_On_1"; L2_Off_1 "Lamp_2_Off_1"; L2_On_2 "Lamp_2_On_2"; L2_Off_2 "Lamp_2_Off_2"; K_L5_W "Light_5_W"; K_L5_On_1 "Light_5_On_a"; K_L5_Off_1 "Light_5_Off_a"; K_L5_On_2 "Light_5_On_b"; K_L5_Off_2 "Light_5_Off_b"; L3_On_1 "Lamp_3_On_1"; L3_Off_1 "Lamp_3_Off_1"; L3_On_2 "Lamp_3_On_2"; L3_Off_2 "Lamp_3_Off_2"; K_L6_W "Light_6_W"; K_L6_On_1 "Light_6_On_a"; K_L6_Off_1 "Light_6_Off_a"
      mask DialogControl Container4 Prompt: House 1
      mask DialogControl Container10 Prompt: Kitchen
      mask DialogControl Container22 Prompt: Bathroom
      mask DialogControl Container20 Prompt: Bedroom 1
      mask DialogControl Container16 Prompt: Bedroom 2
      mask DialogControl Container11 Prompt: Lounge
      mask Display: image('house.jpg');
  House 4 W3 : Subsystem  Commented=on  AncestorBlock=Microgrid_Library/House 4 W  mask{V=240, t=60, K_L1_W=60, K_L1_On_1=69180, K_L1_Off_1=70200, K_L1_On_2=0, K_L1_Off_2=0, K_L2_W=1, K_L2_On_1=0, K_L2_Off_1=0, Fridge_W=150, T_Initial=1, T_Low=1, T_High=3.6, Jug_W=1800, Jug_On_1=23760, Jug_On_2=79800, Jug_On_3=0, Toaster_W=1000, Toaster_On_1=21600, Toaster_On_2=0, N_Elements=2, Oven_On_1=69240, Oven_Off_1=70140, Shower_On_a=20040, Shower_L_a=180, Shower_On_b=0, Shower_L_b=0, Shower_On_c=0, Shower_L_c=0, K_L3_W=40, K_L3_On_1=19800, K_L3_Off_1=20400, K_L3_On_2=0, K_L3_Off_2=0, HW_W=2000, M=88, D=0.488, L=0.955, Ti=7, Ta=20, T_Low_WH=55, T_High_WH=59.5, Clock_1_W=0, Lamp_1_W=1, L1_On_1=0, L1_Off_1=0, L1_On_2=0, L1_Off_2=0, K_L4_W=1, K_L4_On_1=0, K_L4_Off_1=0, Clock_2_W=4, Lamp_2_W=40, L2_On_1=19680, L2_Off_1=21600, L2_On_2=82800, L2_Off_2=84600, K_L5_W=1, K_L5_On_1=0, K_L5_Off_1=0, K_L5_On_2=0, K_L5_Off_2=0, Phone_C_1_W=5, Phone_C_1_On_a=0, Phone_C_1_Off_a=27300, Phone_C_1_On_b=79200, Phone_C_1_Off_b=86400, Phone_C_2_W=0, Phone_C_2_On_a=0, Phone_C_2_Off_a=0, Phone_C_2_On_b=0, Phone_C_2_Off_b=0, Phone_C_3_W=0, Phone_C_3_On_a=0, Phone_C_3_Off_a=0, Phone_C_3_On_b=0, Phone_C_3_Off_b=0, Laptop_C_1_W=35, Laptop_C_1_On_a=63900, Laptop_C_1_Off_a=75600, Laptop_C_2_W=65, Laptop_C_2_On_a=0, Laptop_C_2_Off_a=21600, Laptop_C_2_On_b=66600, Laptop_C_2_Off_b=86400, Lamp_3_W=18, L3_On_1=66000, L3_Off_1=82800, L3_On_2=0, L3_Off_2=0, K_L6_W=40, K_L6_On_1=63000, K_L6_Off_1=66000, Heater_W=2000, Heater_On_1=65100, Heater_Off_1=82200, Stereo_W=100, Stereo_On_1=68640, Stereo_Off_1=70740, TV_W=300, TV_On_1=70800, TV_Off_1=82800, TV_On_2=0, TV_Off_2=0}
      mask prompts: V "Voltage"; t "Time"; K_L1_W "Light_1_W"; K_L1_On_1 "Light_1_On_a"; K_L1_Off_1 "Light_1_Off_a"; K_L1_On_2 "Light_1_On_b"; K_L1_Off_2 "Light_1_Off_b"; K_L2_W "Light_2_W"; K_L2_On_1 "Light_2_On_a"; K_L2_Off_1 "Light_2_Off_a"; T_Initial "Fridge_Initial_Temp"; T_Low "Fridge_T_Low"; T_High "Fridge_T_High"; N_Elements "Oven_#_Elements"; Shower_L_a "Shower_Length_a"; Shower_L_b "Shower_Length_b"; Shower_L_c "Shower_Length_c"; K_L3_W "Light_3_W"; K_L3_On_1 "Light_3_On_a"; K_L3_Off_1 "Light_3_Off_a"; K_L3_On_2 "Light_3_On_b"; K_L3_Off_2 "Light_3_Off_b"; M "Mass of water"; D "HW_Diameter"; L "HW_Length"; Ti "Inlet Temp"; Ta "Ambient Temp"; L1_On_1 "Lamp_1_On_1"; L1_Off_1 "Lamp_1_Off_1"; L1_On_2 "Lamp_1_On_2"; L1_Off_2 "Lamp_1_Off_2"; K_L4_W "Light_4_W"; K_L4_On_1 "Light_4_On_a"; K_L4_Off_1 "Light_4_Off_a"; L2_On_1 "Lamp_2_On_1"; L2_Off_1 "Lamp_2_Off_1"; L2_On_2 "Lamp_2_On_2"; L2_Off_2 "Lamp_2_Off_2"; K_L5_W "Light_5_W"; K_L5_On_1 "Light_5_On_a"; K_L5_Off_1 "Light_5_Off_a"; K_L5_On_2 "Light_5_On_b"; K_L5_Off_2 "Light_5_Off_b"; L3_On_1 "Lamp_3_On_1"; L3_Off_1 "Lamp_3_Off_1"; L3_On_2 "Lamp_3_On_2"; L3_Off_2 "Lamp_3_Off_2"; K_L6_W "Light_6_W"; K_L6_On_1 "Light_6_On_a"; K_L6_Off_1 "Light_6_Off_a"
      mask DialogControl Container4 Prompt: House 1
      mask DialogControl Container10 Prompt: Kitchen
      mask DialogControl Container22 Prompt: Bathroom
      mask DialogControl Container20 Prompt: Bedroom 1
      mask DialogControl Container16 Prompt: Bedroom 2
      mask DialogControl Container11 Prompt: Lounge
      mask Display: image('house.jpg');
  House 5 W1 : Subsystem  AncestorBlock=Microgrid_Library/House 5 W  mask{V=240, t=60, K_L1_W=18, K_L1_On_1=23220, K_L1_Off_1=27120, K_L1_On_2=74160, K_L1_Off_2=82020, Dishwasher_W=1200, Dishwasher_On=36420, Fridge_W=150, T_Initial=1.35, T_Low=1.2, T_High=3.1, Jug_W=1500, Jug_On_1=25620, Jug_On_2=0, Jug_On_3=0, Toaster_W=1100, Toaster_On_1=30600, Toaster_On_2=0, N_Elements=4, Oven_On_1=65040, Oven_Off_1=69900, Shower_On_a=29100, Shower_L_a=240, Shower_On_b=39000, Shower_L_b=300, Shower_On_c=0, Shower_L_c=0, K_L3_W=18, K_L3_On_1=28800, K_L3_Off_1=29400, K_L3_On_2=38700, K_L3_Off_2=39120, HW_W=2000, M=135, D=0.488, L=1.35, Ti=7, Ta=20, T_Low_WH=56, T_High_WH=58, Clock_1_W=3, Lamp_1_W=18, L1_On_1=70560, L1_Off_1=82920, L1_On_2=0, L1_Off_2=0, K_L4_W=40, K_L4_On_1=65400, K_L4_Off_1=76200, Clock_2_W=5, Lamp_2_W=18, L2_On_1=26640, L2_Off_1=29520, L2_On_2=66000, L2_Off_2=79560, K_L5_W=60, K_L5_On_1=77100, K_L5_Off_1=79560, K_L5_On_2=0, K_L5_Off_2=0, Phone_C_1_W=5, Phone_C_1_On_a=0, Phone_C_1_Off_a=8760, Phone_C_1_On_b=77100, Phone_C_1_Off_b=86400, Phone_C_2_W=6, Phone_C_2_On_a=0, Phone_C_2_Off_a=21600, Phone_C_2_On_b=77100, Phone_C_2_Off_b=86400, Phone_C_3_W=5, Phone_C_3_On_a=0, Phone_C_3_Off_a=14820, Phone_C_3_On_b=77100, Phone_C_3_Off_b=86400, Laptop_C_1_W=65, Laptop_C_1_On_a=34200, Laptop_C_1_Off_a=52200, Laptop_C_2_W=65, Laptop_C_2_On_a=72780, Laptop_C_2_Off_a=77100, Laptop_C_2_On_b=0, Laptop_C_2_Off_b=0, Lamp_3_W=24, L3_On_1=25200, L3_Off_1=27000, L3_On_2=20040, L3_Off_2=84000, K_L6_W=100, K_L6_On_1=70200, K_L6_Off_1=73800, Heater_W=2000, Heater_On_1=29160, Heater_Off_1=76140, Stereo_W=50, Stereo_On_1=43560, Stereo_Off_1=45480, TV_W=200, TV_On_1=39900, TV_Off_1=52200, TV_On_2=69600, TV_Off_2=77100}
      mask prompts: V "Voltage"; t "Time"; K_L1_W "Light_1_W"; K_L1_On_1 "Light_1_On_a"; K_L1_Off_1 "Light_1_Off_a"; K_L1_On_2 "Light_1_On_b"; K_L1_Off_2 "Light_1_Off_b"; T_Initial "Fridge_Initial_Temp"; T_Low "Fridge_T_Low"; T_High "Fridge_T_High"; N_Elements "Oven_#_Elements"; Shower_L_a "Shower_Length_a"; Shower_L_b "Shower_Length_b"; Shower_L_c "Shower_Length_c"; K_L3_W "Light_3_W"; K_L3_On_1 "Light_3_On_a"; K_L3_Off_1 "Light_3_Off_a"; K_L3_On_2 "Light_3_On_b"; K_L3_Off_2 "Light_3_Off_b"; M "Mass of water"; D "HW_Diameter"; L "HW_Length"; Ti "Inlet Temp"; Ta "Ambient Temp"; L1_On_1 "Lamp_1_On_1"; L1_Off_1 "Lamp_1_Off_1"; L1_On_2 "Lamp_1_On_2"; L1_Off_2 "Lamp_1_Off_2"; K_L4_W "Light_4_W"; K_L4_On_1 "Light_4_On_a"; K_L4_Off_1 "Light_4_Off_a"; L2_On_1 "Lamp_2_On_1"; L2_Off_1 "Lamp_2_Off_1"; L2_On_2 "Lamp_2_On_2"; L2_Off_2 "Lamp_2_Off_2"; K_L5_W "Light_5_W"; K_L5_On_1 "Light_5_On_a"; K_L5_Off_1 "Light_5_Off_a"; K_L5_On_2 "Light_5_On_b"; K_L5_Off_2 "Light_5_Off_b"; L3_On_1 "Lamp_3_On_1"; L3_Off_1 "Lamp_3_Off_1"; L3_On_2 "Lamp_3_On_2"; L3_Off_2 "Lamp_3_Off_2"; K_L6_W "Light_6_W"; K_L6_On_1 "Light_6_On_a"; K_L6_Off_1 "Light_6_Off_a"
      mask DialogControl Container4 Prompt: House 1
      mask DialogControl Container10 Prompt: Kitchen
      mask DialogControl Container22 Prompt: Bathroom
      mask DialogControl Container20 Prompt: Bedroom 1
      mask DialogControl Container16 Prompt: Bedroom 2
      mask DialogControl Container11 Prompt: Lounge
      mask Display: image('house.jpg');
  House 5 W2 : Subsystem  Commented=on  AncestorBlock=Microgrid_Library/House 5 W  mask{V=240, t=60, K_L1_W=18, K_L1_On_1=23220, K_L1_Off_1=27120, K_L1_On_2=74160, K_L1_Off_2=82020, Dishwasher_W=1200, Dishwasher_On=36420, Fridge_W=150, T_Initial=1.35, T_Low=1.2, T_High=3.1, Jug_W=1500, Jug_On_1=25620, Jug_On_2=0, Jug_On_3=0, Toaster_W=1100, Toaster_On_1=30600, Toaster_On_2=0, N_Elements=4, Oven_On_1=65040, Oven_Off_1=69900, Shower_On_a=29100, Shower_L_a=240, Shower_On_b=39000, Shower_L_b=300, Shower_On_c=0, Shower_L_c=0, K_L3_W=18, K_L3_On_1=28800, K_L3_Off_1=29400, K_L3_On_2=38700, K_L3_Off_2=39120, HW_W=2000, M=135, D=0.488, L=1.35, Ti=7, Ta=20, T_Low_WH=56, T_High_WH=58, Clock_1_W=3, Lamp_1_W=18, L1_On_1=70560, L1_Off_1=82920, L1_On_2=0, L1_Off_2=0, K_L4_W=40, K_L4_On_1=65400, K_L4_Off_1=76200, Clock_2_W=5, Lamp_2_W=18, L2_On_1=26640, L2_Off_1=29520, L2_On_2=66000, L2_Off_2=79560, K_L5_W=60, K_L5_On_1=77100, K_L5_Off_1=79560, K_L5_On_2=0, K_L5_Off_2=0, Phone_C_1_W=5, Phone_C_1_On_a=0, Phone_C_1_Off_a=8760, Phone_C_1_On_b=77100, Phone_C_1_Off_b=86400, Phone_C_2_W=6, Phone_C_2_On_a=0, Phone_C_2_Off_a=21600, Phone_C_2_On_b=77100, Phone_C_2_Off_b=86400, Phone_C_3_W=5, Phone_C_3_On_a=0, Phone_C_3_Off_a=14820, Phone_C_3_On_b=77100, Phone_C_3_Off_b=86400, Laptop_C_1_W=65, Laptop_C_1_On_a=34200, Laptop_C_1_Off_a=52200, Laptop_C_2_W=65, Laptop_C_2_On_a=72780, Laptop_C_2_Off_a=77100, Laptop_C_2_On_b=0, Laptop_C_2_Off_b=0, Lamp_3_W=24, L3_On_1=25200, L3_Off_1=27000, L3_On_2=20040, L3_Off_2=84000, K_L6_W=100, K_L6_On_1=70200, K_L6_Off_1=73800, Heater_W=2000, Heater_On_1=29160, Heater_Off_1=76140, Stereo_W=50, Stereo_On_1=43560, Stereo_Off_1=45480, TV_W=200, TV_On_1=39900, TV_Off_1=52200, TV_On_2=69600, TV_Off_2=77100}
      mask prompts: V "Voltage"; t "Time"; K_L1_W "Light_1_W"; K_L1_On_1 "Light_1_On_a"; K_L1_Off_1 "Light_1_Off_a"; K_L1_On_2 "Light_1_On_b"; K_L1_Off_2 "Light_1_Off_b"; T_Initial "Fridge_Initial_Temp"; T_Low "Fridge_T_Low"; T_High "Fridge_T_High"; N_Elements "Oven_#_Elements"; Shower_L_a "Shower_Length_a"; Shower_L_b "Shower_Length_b"; Shower_L_c "Shower_Length_c"; K_L3_W "Light_3_W"; K_L3_On_1 "Light_3_On_a"; K_L3_Off_1 "Light_3_Off_a"; K_L3_On_2 "Light_3_On_b"; K_L3_Off_2 "Light_3_Off_b"; M "Mass of water"; D "HW_Diameter"; L "HW_Length"; Ti "Inlet Temp"; Ta "Ambient Temp"; L1_On_1 "Lamp_1_On_1"; L1_Off_1 "Lamp_1_Off_1"; L1_On_2 "Lamp_1_On_2"; L1_Off_2 "Lamp_1_Off_2"; K_L4_W "Light_4_W"; K_L4_On_1 "Light_4_On_a"; K_L4_Off_1 "Light_4_Off_a"; L2_On_1 "Lamp_2_On_1"; L2_Off_1 "Lamp_2_Off_1"; L2_On_2 "Lamp_2_On_2"; L2_Off_2 "Lamp_2_Off_2"; K_L5_W "Light_5_W"; K_L5_On_1 "Light_5_On_a"; K_L5_Off_1 "Light_5_Off_a"; K_L5_On_2 "Light_5_On_b"; K_L5_Off_2 "Light_5_Off_b"; L3_On_1 "Lamp_3_On_1"; L3_Off_1 "Lamp_3_Off_1"; L3_On_2 "Lamp_3_On_2"; L3_Off_2 "Lamp_3_Off_2"; K_L6_W "Light_6_W"; K_L6_On_1 "Light_6_On_a"; K_L6_Off_1 "Light_6_Off_a"
      mask DialogControl Container4 Prompt: House 1
      mask DialogControl Container10 Prompt: Kitchen
      mask DialogControl Container22 Prompt: Bathroom
      mask DialogControl Container20 Prompt: Bedroom 1
      mask DialogControl Container16 Prompt: Bedroom 2
      mask DialogControl Container11 Prompt: Lounge
      mask Display: image('house.jpg');
  House 5 W3 : Subsystem  Commented=on  AncestorBlock=Microgrid_Library/House 5 W  mask{V=240, t=60, K_L1_W=18, K_L1_On_1=23220, K_L1_Off_1=27120, K_L1_On_2=74160, K_L1_Off_2=82020, Dishwasher_W=1200, Dishwasher_On=36420, Fridge_W=150, T_Initial=1.35, T_Low=1.2, T_High=3.1, Jug_W=1500, Jug_On_1=25620, Jug_On_2=0, Jug_On_3=0, Toaster_W=1100, Toaster_On_1=30600, Toaster_On_2=0, N_Elements=4, Oven_On_1=65040, Oven_Off_1=69900, Shower_On_a=29100, Shower_L_a=240, Shower_On_b=39000, Shower_L_b=300, Shower_On_c=0, Shower_L_c=0, K_L3_W=18, K_L3_On_1=28800, K_L3_Off_1=29400, K_L3_On_2=38700, K_L3_Off_2=39120, HW_W=2000, M=135, D=0.488, L=1.35, Ti=7, Ta=20, T_Low_WH=56, T_High_WH=58, Clock_1_W=3, Lamp_1_W=18, L1_On_1=70560, L1_Off_1=82920, L1_On_2=0, L1_Off_2=0, K_L4_W=40, K_L4_On_1=65400, K_L4_Off_1=76200, Clock_2_W=5, Lamp_2_W=18, L2_On_1=26640, L2_Off_1=29520, L2_On_2=66000, L2_Off_2=79560, K_L5_W=60, K_L5_On_1=77100, K_L5_Off_1=79560, K_L5_On_2=0, K_L5_Off_2=0, Phone_C_1_W=5, Phone_C_1_On_a=0, Phone_C_1_Off_a=8760, Phone_C_1_On_b=77100, Phone_C_1_Off_b=86400, Phone_C_2_W=6, Phone_C_2_On_a=0, Phone_C_2_Off_a=21600, Phone_C_2_On_b=77100, Phone_C_2_Off_b=86400, Phone_C_3_W=5, Phone_C_3_On_a=0, Phone_C_3_Off_a=14820, Phone_C_3_On_b=77100, Phone_C_3_Off_b=86400, Laptop_C_1_W=65, Laptop_C_1_On_a=34200, Laptop_C_1_Off_a=52200, Laptop_C_2_W=65, Laptop_C_2_On_a=72780, Laptop_C_2_Off_a=77100, Laptop_C_2_On_b=0, Laptop_C_2_Off_b=0, Lamp_3_W=24, L3_On_1=25200, L3_Off_1=27000, L3_On_2=20040, L3_Off_2=84000, K_L6_W=100, K_L6_On_1=70200, K_L6_Off_1=73800, Heater_W=2000, Heater_On_1=29160, Heater_Off_1=76140, Stereo_W=50, Stereo_On_1=43560, Stereo_Off_1=45480, TV_W=200, TV_On_1=39900, TV_Off_1=52200, TV_On_2=69600, TV_Off_2=77100}
      mask prompts: V "Voltage"; t "Time"; K_L1_W "Light_1_W"; K_L1_On_1 "Light_1_On_a"; K_L1_Off_1 "Light_1_Off_a"; K_L1_On_2 "Light_1_On_b"; K_L1_Off_2 "Light_1_Off_b"; T_Initial "Fridge_Initial_Temp"; T_Low "Fridge_T_Low"; T_High "Fridge_T_High"; N_Elements "Oven_#_Elements"; Shower_L_a "Shower_Length_a"; Shower_L_b "Shower_Length_b"; Shower_L_c "Shower_Length_c"; K_L3_W "Light_3_W"; K_L3_On_1 "Light_3_On_a"; K_L3_Off_1 "Light_3_Off_a"; K_L3_On_2 "Light_3_On_b"; K_L3_Off_2 "Light_3_Off_b"; M "Mass of water"; D "HW_Diameter"; L "HW_Length"; Ti "Inlet Temp"; Ta "Ambient Temp"; L1_On_1 "Lamp_1_On_1"; L1_Off_1 "Lamp_1_Off_1"; L1_On_2 "Lamp_1_On_2"; L1_Off_2 "Lamp_1_Off_2"; K_L4_W "Light_4_W"; K_L4_On_1 "Light_4_On_a"; K_L4_Off_1 "Light_4_Off_a"; L2_On_1 "Lamp_2_On_1"; L2_Off_1 "Lamp_2_Off_1"; L2_On_2 "Lamp_2_On_2"; L2_Off_2 "Lamp_2_Off_2"; K_L5_W "Light_5_W"; K_L5_On_1 "Light_5_On_a"; K_L5_Off_1 "Light_5_Off_a"; K_L5_On_2 "Light_5_On_b"; K_L5_Off_2 "Light_5_Off_b"; L3_On_1 "Lamp_3_On_1"; L3_Off_1 "Lamp_3_Off_1"; L3_On_2 "Lamp_3_On_2"; L3_Off_2 "Lamp_3_Off_2"; K_L6_W "Light_6_W"; K_L6_On_1 "Light_6_On_a"; K_L6_Off_1 "Light_6_Off_a"
      mask DialogControl Container4 Prompt: House 1
      mask DialogControl Container10 Prompt: Kitchen
      mask DialogControl Container22 Prompt: Bathroom
      mask DialogControl Container20 Prompt: Bedroom 1
      mask DialogControl Container16 Prompt: Bedroom 2
      mask DialogControl Container11 Prompt: Lounge
      mask Display: image('house.jpg');
  Integrator{1..2,5..6} (4 alike) : Integrator  Commented=on
  Integrator3 : Integrator
  Integrator4 : Integrator
  Mux1 : Mux
  Mux10 : Mux  Commented=on
  Mux11 : Mux  Commented=on  Inputs=2
  Mux12 : Mux  Inputs=3
  Mux2 : Mux  Commented=on  Inputs=3
  Mux3 : Mux  Inputs=2
  Mux4 : Mux  Inputs=3
  Mux5 : Mux  Commented=on  Inputs=2
  Mux6 : Mux  Commented=on
  Mux7 : Mux  Commented=on  Inputs=2
  Mux8 : Mux  Commented=on  Inputs=3
  Mux9 : Mux  Commented=on  Inputs=3
  PV1 : Microgrid_Library/PV  P=52
  PV2 : Microgrid_Library/PV  Commented=on  P=52
  PV3 : Microgrid_Library/PV  Commented=on  P=52
  Scope1 : Scope
  Scope2 : Scope  Commented=on
  Scope3 : Scope  NumInputPorts=2
  Scope4 : Scope  NumInputPorts=3
  Scope5 : Scope  Commented=on  NumInputPorts=2
  Scope6 : Scope  Commented=on  NumInputPorts=3
  Scope7 : Scope  Commented=on
  Scope8 : Scope  Commented=on  NumInputPorts=2
  Scope9 : Scope  Commented=on  NumInputPorts=3
  Sum : Sum  Inputs=|+-+|
  Sum1 : Sum  Inputs=++++
  Sum{2..3,5..7} (5 alike) : Sum  Commented=on  Inputs=++++
  Sum4 : Sum  Inputs=++++
  Sum8 : Sum  Commented=on  Inputs=|+-
  Total WH Power : Sum  Commented=on  Inputs=++++
  Total WH Power1 : Sum  Inputs=++++
  Unused Solar : Sum  Commented=on  Inputs=-+|
  WH Powers1 : Mux  Commented=on
  WH Powers2 : Mux  Commented=on
  WH Powers3 : Mux
  WH Temps1 : Mux  Commented=on
  WH Temps2 : Mux  Commented=on
  WH Temps3 : Mux
  WH_Helper_H1 : Subsystem  Commented=on
  WH_Helper_H2 : Subsystem  Commented=on
  WH_Helper_H3 : Subsystem
  powergui : powerlib/powergui  Priority=1  SimulationMode=Continuous  SampleTime=50e-6  frequency=60  Iterations=50  frequencyindice=0  Pbase=100e6  ErrMax=1e-4  UnitsV=kV  UnitsW=MW  buscounter=0  FunctionMessages=off  echomessages=off  EnableUseOfTLC=off  CurrentSourceSwitches=off  DisableSnubberDevices=off  DisableRonSwitches=off  DisableVfSwitches=off  DisplayEquations=off  AutomaticDiscreteSolvers=off  SolverType=Tustin/Backward Euler (TBE)  Interpol=off  ExternalGateDelay=off  methode=off  Ts=100  x0status=blocks  SPID=on  SwTol=0  HookPort=off  NonlinearTolerance=1e-4  nMaxIteration=100  ContinueOnMaxIteration=off  RestoreLinks=warning  ResistiveCurrentMeasurement=off  Frange=[0:2:500]  Ylog=off  Xlog=on  ShowGrid=off  save=off  variable=ZData  structure=0  ZoomFFT=off  StartTime=0.0  cycles=1  DisplayStyle=1  fundamental=60  FreqAxis=off  MaxFrequency=1000  frequencyindicesteady=1  RmsSteady=1  display=off
  unserviced (%)1 : Display
  unserviced (%)2 : Display  Commented=on
  unserviced (%)3 : Display  Commented=on
  wires:
  House 3 W2/1(House 3 House Power) -> Sum2/2
  Clock2/1 -> Gain3/1
  Integrator1/1 -> Divide2/1
  Gain4/1 -> unserviced (%)2/1
  Mux2/1 -> Scope2/1
  WH_Helper_H1/1(WH Bat) -> Mux2/1
  WH Temps1/1 -> Scope6/3
  House 3 W2/3(House 3 WH Temp) -> WH Temps1/2
  1-D Lookup Table2/1 -> PV2/1
  House 5 W2/1(House 5 House Power) -> Sum2/4
  WH_Helper_H1/2(House Bat) -> Mux2/2
  PV2/1 -> Mux5/1
  PV2/2 -> Mux5/2
  BMS2/1 -> PV2/2
  House 5 W2/3(House 5 WH Temp) -> WH Temps1/4
  WH_Helper_H1/3(WH Solar) -> Mux2/3
  House 2 W2/3(House 2 WH Temp) -> WH Temps1/1
  BMS2/7 -> Goto3/1
  Sum2/1 -> WH_Helper_H1/1(House P)
  Divide2/1 -> Gain4/1
  Mux6/1 -> Scope5/2
  WH Powers1/1 -> Scope6/2
  House 4 W2/1(House 4 House Power) -> Sum2/3
  BMS2/4 -> Integrator1/1, Mux6/2
  Gain3/1 -> 1-D Lookup Table2/1
  BMS2/5 -> Mux6/3
  Mux5/1 -> Goto2/1, Scope5/1
  BMS2/3 -> Mux6/1
  BMS2/6 -> Integrator2/1, Mux6/4
  From3/1 -> WH_Helper_H1/3("BMS Bat Supply ")
  Integrator2/1 -> Divide2/2
  House 4 W2/3(House 4 WH Temp) -> WH Temps1/3
  House 2 W2/1(House 2 House Power) -> Sum2/1
  From1/1 -> Mux11/2
  Sum3/1 -> WH_Helper_H1/2(WH P)
  Total WH Power/1 -> Mux7/1
  Mux7/1 -> Scope9/1
  Sum5/1 -> WH_Helper_H2/1(House P)
  Sum6/1 -> WH_Helper_H2/2(WH P)
  House 5 W3/1(House 5 House Power) -> Sum5/4
  House 4 W3/1(House 4 House Power) -> Sum5/3
  House 3 W3/1(House 3 House Power) -> Sum5/2
  House 2 W3/1(House 2 House Power) -> Sum5/1
  Mux8/1 -> Scope7/1
  From5/1 -> WH_Helper_H2/3("BMS Bat Supply ")
  BMS3/7 -> Goto5/1
  From4/1 -> Mux7/2
  WH_Helper_H2/3(WH Solar) -> Sum8/2, Mux8/3
  WH_Helper_H2/1(WH Bat) -> Mux8/1
  WH_Helper_H2/2(House Bat) -> Mux8/2
  WH Temps2/1 -> Scope9/3
  House 5 W3/3(House 5 WH Temp) -> WH Temps2/4
  House 4 W3/3(House 4 WH Temp) -> WH Temps2/3
  House 3 W3/3(House 3 WH Temp) -> WH Temps2/2
  House 2 W3/3(House 2 WH Temp) -> WH Temps2/1
  Divide3/1 -> Gain6/1
  Mux10/1 -> Scope8/2
  WH Powers2/1 -> Scope9/2
  House 2 W3/2(House 2 WH Power) -> WH Powers2/1, Total WH Power/1, Sum6/1
  Gain6/1 -> unserviced (%)3/1
  Clock3/1 -> Gain5/1
  BMS3/4 -> Mux10/2, Integrator5/1
  BMS3/5 -> Mux10/3
  Mux9/1 -> Goto4/1, Scope8/1
  Gain5/1 -> 1-D Lookup Table3/1
  Integrator6/1 -> Divide3/2
  Integrator5/1 -> Divide3/1
  BMS3/3 -> Mux10/1
  BMS3/6 -> Mux10/4, Integrator6/1
  PV3/2 -> Sum8/1, Mux9/2
  BMS3/1 -> PV3/2
  House 4 W3/2(House 4 WH Power) -> Sum6/3, Total WH Power/3, WH Powers2/3
  1-D Lookup Table3/1 -> PV3/1
  House 5 W3/2(House 5 WH Power) -> Total WH Power/4, WH Powers2/4, Sum6/4
  House 3 W3/2(House 3 WH Power) -> Sum6/2, Total WH Power/2, WH Powers2/2
  PV3/1 -> Mux9/1, Unused Solar/2
  Sum8/1 -> Unused Solar/1
  Unused Solar/1 -> House 5 W3/1(unused_solar), House 4 W3/1(unused_solar), House 3 W3/1(unused_solar), House 2 W3/1(unused_solar), Mux9/3
  House 3 W2/2(House 3 WH Power) -> Sum3/2, WH Powers1/2, Sum7/2
  House 2 W2/2(House 2 WH Power) -> Sum3/1, Sum7/1, WH Powers1/1
  House 4 W2/2(House 4 WH Power) -> WH Powers1/3, Sum7/3, Sum3/3
  House 5 W2/2(House 5 WH Power) -> Sum3/4, WH Powers1/4, Sum7/4
  Mux11/1 -> Scope6/1
  Sum7/1 -> Mux11/1
  PV1/1 -> Mux12/1, Sum/1
  House 3 W1/2(House 3 WH Power) -> WH Powers3/2, Total WH Power1/2, Sum4/2
  House 5 W1/2(House 5 WH Power) -> Sum4/4, WH Powers3/4, Total WH Power1/4
  1-D Lookup Table1/1 -> PV1/1
  House 4 W1/2(House 4 WH Power) -> WH Powers3/3, Total WH Power1/3, Sum4/3
  BMS1/1 -> PV1/2
  PV1/2 -> Sum/2, Mux12/2
  BMS1/6 -> Integrator4/1, Mux1/4
  BMS1/3 -> Mux1/1
  Integrator3/1 -> Divide1/1
  Integrator4/1 -> Divide1/2
  Gain1/1 -> 1-D Lookup Table1/1
  Mux12/1 -> Scope3/1, [PV_MUX]
  BMS1/5 -> Mux1/3
  BMS1/4 -> Integrator3/1, Mux1/2
  Clock1/1 -> Gain1/1
  Gain2/1 -> unserviced (%)1/1
  House 2 W1/2(House 2 WH Power) -> Sum4/1, Total WH Power1/1, WH Powers3/1
  WH Powers3/1 -> Scope4/2
  Mux1/1 -> Scope3/2
  Divide1/1 -> Gain2/1
  House 2 W1/3(House 2 WH Temp) -> WH Temps3/1
  House 3 W1/3(House 3 WH Temp) -> WH Temps3/2
  House 4 W1/3(House 4 WH Temp) -> WH Temps3/3
  House 5 W1/3(House 5 WH Temp) -> WH Temps3/4
  WH Temps3/1 -> Scope4/3
  WH_Helper_H3/2(House Bat) -> Mux4/2
  WH_Helper_H3/1(WH Bat) -> Mux4/1
  WH_Helper_H3/3(WH Solar) -> Sum/3, Mux4/3
  [PV_MUX] -> Mux3/2
  BMS1/7 -> [bat_sup]
  [bat_sup] -> WH_Helper_H3/3("BMS Bat Supply ")
  Mux4/1 -> Scope1/1
  House 2 W1/1(House 2 House Power) -> Sum1/1
  House 3 W1/1(House 3 House Power) -> Sum1/2
  House 4 W1/1(House 4 House Power) -> Sum1/3
  House 5 W1/1(House 5 House Power) -> Sum1/4
  Sum4/1 -> WH_Helper_H3/2(WH P)
  Sum1/1 -> WH_Helper_H3/1(House P)
  Mux3/1 -> Scope4/1
  Total WH Power1/1 -> Mux3/1
  Sum/1 -> House 2 W1/1(unused_solar), House 5 W1/1(unused_solar), House 4 W1/1(unused_solar), House 3 W1/1(unused_solar)
  connections:
  58m2/RConn1 -- House 4 W2/LConn1 -- 47m2/LConn1
  161m2/RConn1 -- House 2 W2/LConn1 -- 60m2/LConn1
  58m2/LConn1 -- House 3 W2/LConn1 -- 60m2/RConn1
  PV2/RConn1 -- BMS2/RConn1
  47m2/RConn1 -- House 5 W2/LConn1
  BMS2/RConn4 -- 161m2/LConn1
  47m3/LConn1 -- House 4 W3/LConn1 -- 58m3/RConn1
  60m3/RConn1 -- House 3 W3/LConn1 -- 58m3/LConn1
  60m3/LConn1 -- House 2 W3/LConn1 -- 161m3/RConn1
  PV3/RConn1 -- BMS3/RConn1
  BMS3/RConn4 -- 161m3/LConn1
  47m3/RConn1 -- House 5 W3/LConn1
  47m1/LConn1 -- 58m1/RConn1 -- House 4 W1/LConn1
  60m1/RConn1 -- 58m1/LConn1 -- House 3 W1/LConn1
  60m1/LConn1 -- 161m1/RConn1 -- House 2 W1/LConn1
  BMS1/RConn4 -- 161m1/LConn1
  47m1/RConn1 -- House 5 W1/LConn1
  PV1/RConn1 -- BMS1/RConn1
